simulink model "tendon_transmission_system_2018b"  (R2018b)
settings: Solver=VariableStepAuto  StartTime=0.0  StopTime=10.0  RelTol=1e-3
values from neighbouring files (symbols this model uses):
  parameters = [k1, k2, b2, mu_d, mu_s, omega, sigma, b]    [tendon_driven_system.m]
undefined symbols (not defined in the file or in its folder): sigbuilder_block
settings Model: Creator=ge26jow  LastModifiedBy=ge26jow
settings DataIOCC: ReturnWorkspaceOutputs=on
settings DebuggingCC: UnconnectedInputMsg=none  UnconnectedOutputMsg=none  UnconnectedLineMsg=none  SFMachineParentedDataDiag=error
settings ModelReferenceCC: EnableRefExpFcnMdlSchedulingChecks=off
settings RTWCC: Description=Generic Real-Time Target

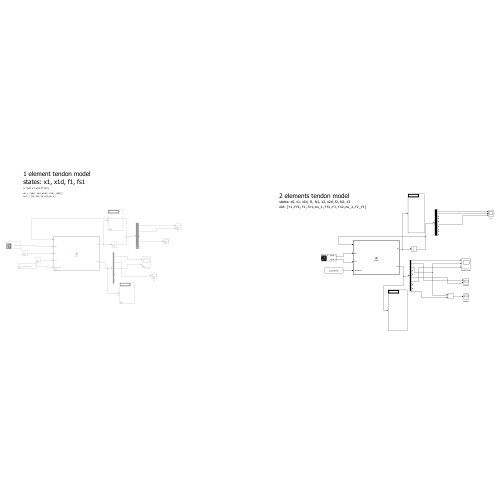
[thumbnail: Simulink's stored preview of the top-level diagram]
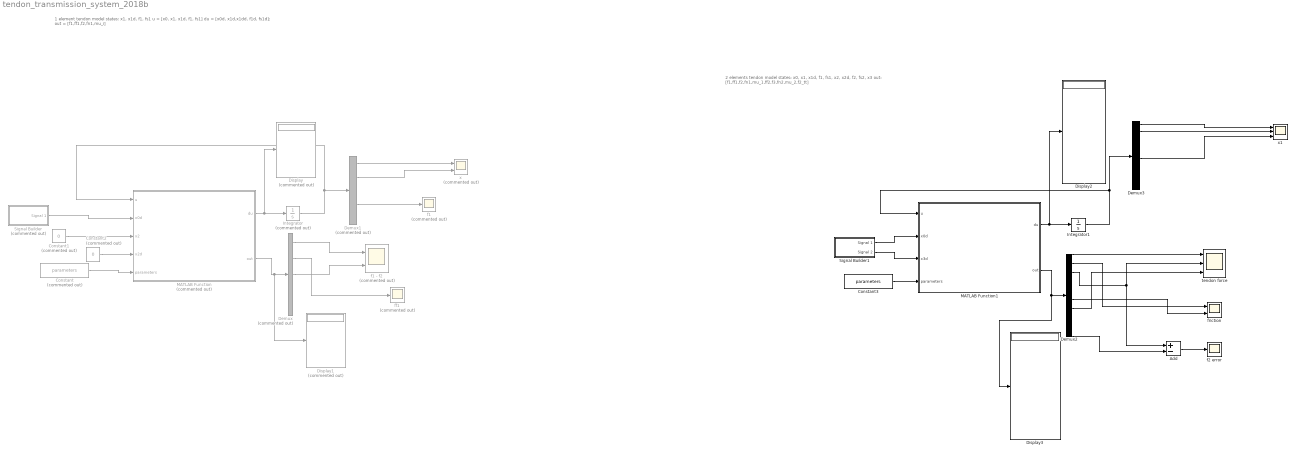
== system tendon_transmission_system_2018b ==
  note: 2 elements tendon model
      | states: x0, x1, x1d, f1, fs1, x2, x2d, f2, fs2, x3
      | out: [f1,ff1,f2,fn1,mu_1,ff2,f3,fn2,mu_2,f2_tt]
  note: 1 element tendon model
      | states: x1, x1d, f1, fs1
      |
      | u = [x0, x1, x1d, f1, fs1]
      |
      | du = [x0d, x1d,x1dd, f1d, fs1d];
      | out = [f1,ff1,f2,fn1,mu_i]
  Add : Sum  Inputs=+-
  Constant : Constant  Commented=on  Value=parameters
  Constant1 : Constant  Commented=on  Value=0
  Constant2 : Constant  Commented=on  Value=0
  Constant3 : Constant  Value=parameters
  Demux : Demux  Commented=on  Outputs=5
  Demux1 : Demux  Commented=on  Outputs=5
  Demux2 : Demux  Outputs=10
  Demux3 : Demux  Outputs=10
  Display : Display  Commented=on
  Display1 : Display  Commented=on
  Display2 : Display
  Display3 : Display
  Integrator : Integrator  Commented=on  InitialCondition=[0,0,0,0,0]
  Integrator1 : Integrator  InitialCondition=[0,0,0,0,0,0,0,0,0,0]
  MATLAB Function : MATLAB Function  Commented=on  TreatAsAtomicUnit=on
  MATLAB Function1 : MATLAB Function  TreatAsAtomicUnit=on
  Signal Builder : Subsystem  Tag=STV Subsys  Commented=on  LoadFcn=sigbuilder_block('load');  StartFcn=sigbuilder_block('start');  StopFcn=sigbuilder_block('stop');  ClipboardFcn=sigbuilder_block('clipboard');  mask(Sigbuilder block){tuvar=[0:10]}
      mask help: Simulink:masks:SigbuilderBlock_MD
      mask init:
      | if ~strcmp(get_param(bdroot(gcbh),'SimulationStatus'),'stopped') tuvar = sigbuilder_block('maskInit'); end
      settings: CopyFcn=sigbuilder_block('copy');  DeleteFcn=sigbuilder_block('delete');  ModelCloseFcn=sigbuilder_block('modelClose');  PreSaveFcn=sigbuilder_block('preSave');  PauseFcn=sigbuilder_block('pause');  ContinueFcn=sigbuilder_block('continue');  NameChangeFcn=sigbuilder_block('namechange');  OpenFcn=sigbuilder_block('open',[437.6 199.2 550.4 400 ]);  CloseFcn=sigbuilder_block('close');
      mask Display: plot(0, 0, 100, 100,[2, 2, 32, 32, 2], [68, 8, 8, 68, 68],[32, 2], [38, 38], [32, 19, 2],[53, 60, 44], [32, 17, 17, 2],[16, 16, 31, 31]);txt = getActiveGroup(gcbh);text(2, 100, txt,'verticalAlignment', 'top');
  Signal Builder1 : Subsystem  Tag=STV Subsys  LoadFcn=sigbuilder_block('load');  StartFcn=sigbuilder_block('start');  StopFcn=sigbuilder_block('stop');  ClipboardFcn=sigbuilder_block('clipboard');  mask(Sigbuilder block){tuvar=[0:10]}
      mask help: Simulink:masks:SigbuilderBlock_MD
      mask init:
      | if ~strcmp(get_param(bdroot(gcbh),'SimulationStatus'),'stopped') tuvar = sigbuilder_block('maskInit'); end
      settings: CopyFcn=sigbuilder_block('copy');  DeleteFcn=sigbuilder_block('delete');  ModelCloseFcn=sigbuilder_block('modelClose');  PreSaveFcn=sigbuilder_block('preSave');  PauseFcn=sigbuilder_block('pause');  ContinueFcn=sigbuilder_block('continue');  NameChangeFcn=sigbuilder_block('namechange');  OpenFcn=sigbuilder_block('open',[393 197.25 550.5 399.75 ]);  CloseFcn=sigbuilder_block('close');
      mask Display: plot(0, 0, 100, 100,[2, 2, 32, 32, 2], [68, 8, 8, 68, 68],[32, 2], [38, 38], [32, 19, 2],[53, 60, 44], [32, 17, 17, 2],[16, 16, 31, 31]);txt = getActiveGroup(gcbh);text(2, 100, txt,'verticalAlignment', 'top');
  f1 : Scope  Commented=on
  f1 - f2 : Scope  Commented=on  NumInputPorts=2
  f2 error : Scope
  ff1 : Scope  Commented=on
  friction : Scope  NumInputPorts=2
  tendon force : Scope  NumInputPorts=3
  x : Scope  Commented=on  NumInputPorts=2
  x1 : Scope  NumInputPorts=3
  wires:
  MATLAB Function/1(du) -> Display/1, Integrator/1
  Integrator/1 -> Demux1/1, MATLAB Function/1(u)
  Constant/1 -> MATLAB Function/5(parameters)
  Constant1/1 -> MATLAB Function/3(x2)
  Constant2/1 -> MATLAB Function/4(x2d)
  Signal Builder/1(Signal 1) -> MATLAB Function/2(x0d)
  MATLAB Function/2(out) -> Display1/1, Demux/1
  Demux1/1 -> x/1
  Demux/1 -> f1 - f2/1
  Demux/3 -> f1 - f2/2
  Demux1/2 -> x/2
  Demux1/4 -> f1/1
  Demux/2 -> ff1/1
  Demux2/3 -> tendon force/2, Add/1
  MATLAB Function1/2(out) -> Display3/1, Demux2/1
  Demux3/2 -> x1/2
  Demux2/2 -> friction/1
  Integrator1/1 -> Demux3/1, MATLAB Function1/1(u)
  Demux2/1 -> tendon force/1
  MATLAB Function1/1(du) -> Display2/1, Integrator1/1
  Constant3/1 -> MATLAB Function1/4(parameters)
  Demux3/1 -> x1/1
  Signal Builder1/1(Signal 1) -> MATLAB Function1/2(x0d)
  Demux2/7 -> tendon force/3
  Demux2/10 -> Add/2
  Add/1 -> f2 error/1
  Demux3/6 -> x1/3
  Demux2/6 -> friction/2
  Signal Builder1/2(Signal 2) -> MATLAB Function1/3(x3d)

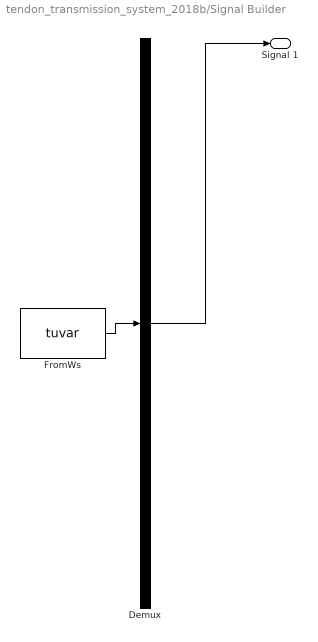
== system tendon_transmission_system_2018b/Signal Builder ==
  Demux : Demux  Tag=STV Demux  Outputs=1
      settings: DisplayOption=none
  FromWs : FromWorkspace  Tag=STV FromWs  VariableName=tuvar
      SigBuilderData=|
      | common.afterFinalStr = 'Extrapolate'
      | common.sampleTime = 0
      | dataSet.timeRange = [0 10]
      | dataSet.name = 'Group 1'
      | sbobj.Groups.Name = 'Group 1'
      | sbobj.Groups.Signals.Name = 'Signal 1'
      | sbobj.Groups.Signals.XData = [0 1 3 4 5 6 7 8 10]
      | sbobj.Groups.Signals.YData = [0 0 0.0005 0.0005 0 0 -0.0009 0 0]
  Signal 1 : Outport  Tag=STV Outport
  wires:
  Demux/1 -> Signal 1/1
  FromWs/1 -> Demux/1

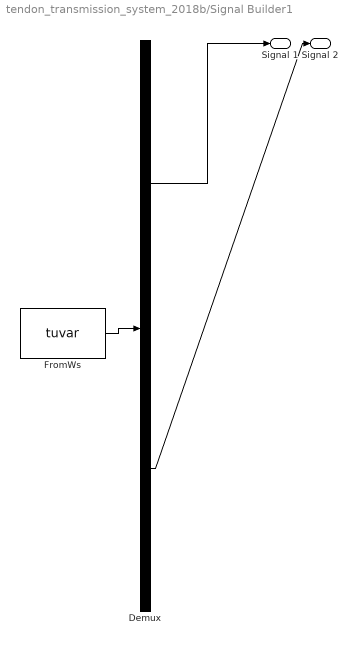
== system tendon_transmission_system_2018b/Signal Builder1 ==
  Demux : Demux  Tag=STV Demux  Outputs=2
      settings: DisplayOption=none
  FromWs : FromWorkspace  Tag=STV FromWs  VariableName=tuvar
      SigBuilderData=|
      | common.afterFinalStr = 'Extrapolate'
      | common.sampleTime = 0
      | dataSet(1).timeRange = [0 10]
      | dataSet(1).name = 'Group 1'
      | dataSet(2).timeRange = [0 10]
      | dataSet(2).name = 'Group 2'
      | sbobj.Groups(1).Name = 'Group 1'
      | sbobj.Groups(1).Signals(1).Name = 'Signal 1'
      | sbobj.Groups(1).Signals(1).XData = [0 1 2 3 4 7 8 9 10]
      | sbobj.Groups(1).Signals(1).YData = [0 0 0.001 0.001 0 0 0 0 0]
      | sbobj.Groups(1).Signals(2).Name = 'Signal 2'
      | sbobj.Groups(1).Signals(2).XData = [0 5 6 6 7 8 8.5 9 10]
      | sbobj.Groups(1).Signals(2).YData = [0 0 -0.001 -0.00101 0 0 0.002 -5e-06 -1e-05]
      | sbobj.Groups(2).Name = 'Group 2'
      | sbobj.Groups(2).Signals(1).Name = 'Signal 1'
      | sbobj.Groups(2).Signals(1).XData = [0 1 2 3 4 6 7 8 9 10]
      | sbobj.Groups(2).Signals(1).YData = [0 0 0.002 0.002 0 0 -0.0015 -0.0015 0 0]
      | sbobj.Groups(2).Signals(2).Name = 'Signal 2'
      | sbobj.Groups(2).Signals(2).XData = [0 5 6 7 8 9 10]
      | sbobj.Groups(2).Signals(2).YData = [0 0 0 0 0 -5e-06 -1e-05]
  Signal 1 : Outport  Tag=STV Outport
  Signal 2 : Outport  Tag=STV Outport  Port=2
  wires:
  Demux/1 -> Signal 1/1
  FromWs/1 -> Demux/1
  Demux/2 -> Signal 2/1

== matlab function tendon_transmission_system_2018b/MATLAB Function1 ==
  data: u input; du output; x0d input; x3d input; parameters input; out output
function [du,out] = dudt(u, x0d, x3d, parameters)
% u = [ x0, x1, x1d, f1, fs1, x2, x2d, f1, fs2, x3 ]
% du = [x0d, x1d, x1dd, f1d, fs1d]
% parameters = [k1, k2, b2, mu_d, mu_s, omega, sigma, b]
x0 = u(1);
x1 = u(2);
x1d = u(3);
f1 = u(4);
fs1 = u(5);
x2 = u(6);
x2d = u(7);
f2 = u(8);
fs2 = u(9);
x3 = u(10);

k1 = parameters(1);
k2 = parameters(2);
b2 = parameters(3);
mu_d = parameters(4);
mu_s = parameters(5);
omega = parameters(6);
sigma = parameters(7);
b = parameters(8);

% element 1
% friction model (f2 is state)
f2_tt = f1 - fs1 - b*x1d;
if x1d == 0
    vs1 = 1;
else 
    vs1 = sign(x1d);
end
% fn1 = f1 + f2;
fn1 = f1*(1+exp(-mu_d*vs1)) + 5;
mu_d1 = abs(1-exp(-mu_d*vs1))/(1+exp(-mu_d*vs1));
mu_s1 = mu_d1*mu_s/mu_d;
mu_1 = mu_d1 + (mu_s1 - mu_d1)*exp(-abs(x1d)/omega);
fs1d = sigma*(x1d-fs1/(fn1*mu_1)*abs(x1d));

ff1 = fs1+b*x1d;
% f1d
f1d = (k1+k2)*(x0d-x1d)+ k1*k2/b2*(x0-x1) - k2/b2*f1;
% if (x0-x1) <= 0
%     f1d = 0;
% end

% x1dd
x1dd = 1/b*(f1d-fs1d + k2/b2*(f1-fs1-b*x1d)- (k1+k2)*(x1d-x2d)- k1*k2/b2*(x1-x2));

% element 2
% friction model
f3 = f2 - fs2 - b*x2d;
if x2d == 0
    vs2 = 1;
else 
    vs2 = sign(x2d);
end
% fn1 = f1 + f2;
fn2 = f2*(1+exp(-mu_d*vs2)) + 5;
mu_d2 = abs(1-exp(-mu_d*vs2))/(1+exp(-mu_d*vs2));
mu_s2 = mu_d2*mu_s/mu_d;
mu_2 = mu_d2 + (mu_s2 - mu_d2)*exp(-abs(x2d)/omega);
fs2d = sigma*(x2d-fs2/(fn2*mu_2)*abs(x2d));

ff2 = fs2+b*x2d;
% f1d
f2d = (k1+k2)*(x1d-x2d)+ k1*k2/b2*(x1-x2) - k2/b2*f2;
% if (x0-x1) <= 0
%     f1d = 0;
% end

% x2dd
x2dd = 1/b*(f2d-fs2d + k2/b2*(f2-fs2-b*x2d)- (k1+k2)*(x2d-x3d)- k1*k2/b2*(x2-x3));

% outputs
du = [x0d, x1d,x1dd, f1d, fs1d, x2d,x2dd, f2d, fs2d, x3d];
out = [f1,ff1,f2,fn1,mu_1,ff2,f3,fn2,mu_2,f2_tt];

== matlab function tendon_transmission_system_2018b/MATLAB Function ==
  data: u input; du output; x0d input; x2 input; x2d input; parameters input; out output
function [du,out] = dudt(u, x0d, x2, x2d, parameters)
% u = [ x0, x1, x1d, f1, fs1]
% du = [x0d, x1d, x1dd, f1d, fs1d]
% out = [f1,ff1,f2,fn1,mu_i];
% parameters = [k1, k2, b2, mu_d, mu_s, omega, sigma, b]
x0 = u(1);
x1 = u(2);
x1d = u(3);
f1 = u(4);
fs1 = u(5);

k1 = parameters(1);
k2 = parameters(2);
b2 = parameters(3);
mu_d = parameters(4);
mu_s = parameters(5);
omega = parameters(6);
sigma = parameters(7);
b = parameters(8);

% friction model
f2 = f1 - fs1 - b*x1d;

if x1d == 0
    vs1 = 1;
else 
    vs1 = sign(x1d);
end
% fn1 = f1 + f2;
fn1 = f1*(1+exp(-mu_d*vs1)) + 5;
mu_di = abs(1-exp(-mu_d*vs1))/(1+exp(-mu_d*vs1));
mu_si = mu_di*mu_s/mu_d;
mu_i = mu_di + (mu_si - mu_di)*exp(-abs(x1d)/omega);
fs1d = sigma*(x1d-fs1/(fn1*mu_i)*abs(x1d));

ff1 = fs1+b*x1d;

% f1d


f1d = (k1+k2)*(x0d-x1d)+ k1*k2/b2*(x0-x1) - k2/b2*f1;
% if (x0-x1) <= 0
%     f1d = 0;
% end

% x1dd

x1dd = 1/b*(f1d-fs1d + k2/b2*(f1-fs1-b*x1d)- (k1+k2)*(x1d-x2d)- k1*k2/b2*(x1-x2));


du = [x0d, x1d,x1dd, f1d, fs1d];
out = [f1,ff1,f2,fn1,mu_i];
